simulink model "SCR_CIRCUIT_"  (R2025a)
settings: Solver=VariableStepAuto  StartTime=0.0  StopTime=10.0  RelTol=1e-3
libraries: spsControlledVoltageSourceLib x1, spsMultimeterLib x1, spsSeriesRLCBranchLib x1, simulink x1, spsThyristorLib x1, sps_lib x1
settings Model: Creator=Admin  LastModifiedBy=samar

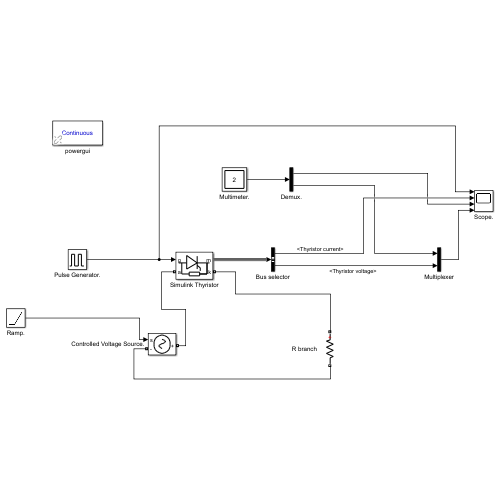
[thumbnail: Simulink's stored preview of the top-level diagram]
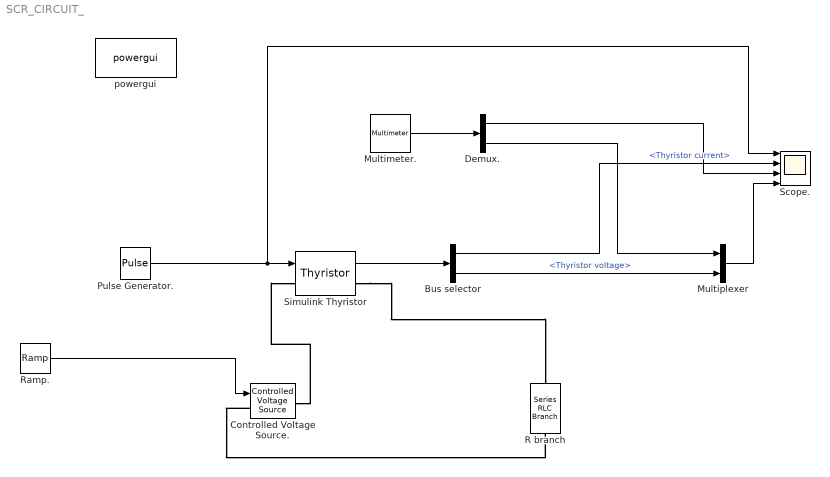
== system SCR_CIRCUIT_ ==
  Bus selector : BusSelector  OutputSignals=Thyristor current,Thyristor voltage
  Controlled Voltage Source. : spsControlledVoltageSourceLib/Controlled Voltage Source  Initialize=on  Source_Type=AC  Amplitude=0  Phase=0  Frequency=0  Measurements=Voltage
  Demux. : Demux  Outputs=2
  Multimeter. : spsMultimeterLib/Multimeter  L=3  sel=[1 2]  yselected={}  Gain=[1 1]  OutputType=Complex  PlotAtSimulationStop=on  PhasorSimulation=off
  Multiplexer : Mux  Inputs=2
  Pulse Generator. : DiscretePulseGenerator  PulseType=Time based  Period=1  PulseWidth=50
  R branch : spsSeriesRLCBranchLib/Series RLC Branch  LConnTagsString=__new0  RConnTagsString=__new0  BranchType=R  Resistance=1  Inductance=1e-3  SetiL0=off  InitialCurrent=0  Capacitance=1e-6  Setx0=off  InitialVoltage=0  Measurements=Branch voltage and current
  Ramp. : simulink/Sources/Ramp  slope=1  start=0  InitialOutput=0
  Scope. : Scope  NumInputPorts=4
      settings: ActiveDisplayYMinimum=-0.12499999999999997  ActiveDisplayYMaximum=1.125
  Simulink Thyristor : spsThyristorLib/Thyristor  Ron=0.001  Lon=0  Vf=0.8  IC=0  Rs=500  Cs=250e-9  Measurements=on
  powergui : sps_lib/powergui  Priority=1  SimulationMode=Continuous  SampleTime=50e-6  frequency=60  Iterations=50  frequencyindice=0  Pbase=100e6  ErrMax=1e-4  UnitsV=kV  UnitsW=MW  buscounter=0  FunctionMessages=off  echomessages=off  EnableUseOfTLC=off  CurrentSourceSwitches=off  DisableSnubberDevices=off  DisableRonSwitches=off  DisableVfSwitches=off  DisplayEquations=off  AutomaticDiscreteSolvers=off  SolverType=Tustin/Backward Euler (TBE)  Interpol=off  ExternalGateDelay=off  methode=off  Ts=100  x0status=blocks  SPID=on  SwTol=0  HookPort=off  NonlinearTolerance=1e-4  nMaxIteration=100  ContinueOnMaxIteration=off  RestoreLinks=warning  ResistiveCurrentMeasurement=off  Frange=[0:2:500]  Ylog=off  Xlog=on  ShowGrid=off  save=off  variable=ZData  structure=0  ZoomFFT=off  StartTime=0.0  cycles=1  DisplayStyle=1  fundamental=60  FreqAxis=off  MaxFrequency=1000  frequencyindicesteady=1  RmsSteady=1  display=off
  wires:
  Pulse Generator./1 -> Scope./1, Simulink Thyristor/1
  Ramp./1 -> Controlled Voltage Source./1
  Simulink Thyristor/1 -> Bus selector/1
  Multimeter./1 -> Demux./1
  Demux./1 -> Scope./3
  Demux./2 -> Multiplexer/1
  Multiplexer/1 -> Scope./4
  Bus selector/2 -> Multiplexer/2  "<Thyristor voltage>"
  Bus selector/1 -> Scope./2  "<Thyristor current>"
  connections:
  Controlled Voltage Source./RConn1 -- Simulink Thyristor/LConn1
  Simulink Thyristor/RConn1 -- R branch/LConn1
  Controlled Voltage Source./LConn1 -- R branch/RConn1
